simulink model "lab7_t24"  (R2021a)
settings: Solver=VariableStepAuto  StartTime=0.0  StopTime=10.0  RelTol=1e-3
libraries: simulink x1
settings Model: Creator=reemb  LastModifiedBy=reemb

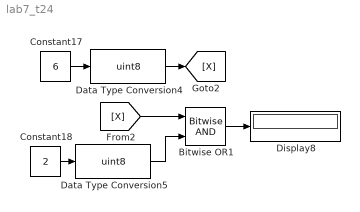
== system lab7_t24 ==
  Bitwise OR1 : simulink/Logic and Bit Operations/Bitwise Operator  logicop=AND  UseBitMask=off  NumInputPorts=2  BitMask=bin2dec('11011001')  BitMaskRealWorld=Stored Integer
  Constant17 : Constant  Value=6
  Constant18 : Constant  Value=2
  Data Type Conversion4 : DataTypeConversion  OutDataTypeStr=uint8  RndMeth=Round
  Data Type Conversion5 : DataTypeConversion  OutDataTypeStr=uint8  RndMeth=Round
  Display8 : Display
  wires:
  [X] -> Bitwise OR1/1
  Data Type Conversion5/1 -> Bitwise OR1/2
  Bitwise OR1/1 -> Display8/1
  Constant18/1 -> Data Type Conversion5/1
  Data Type Conversion4/1 -> [X]
  Constant17/1 -> Data Type Conversion4/1
